simulink model "DOF2_P_SH_ADD_PID_4_0620"  (R2024a)
settings: Solver=ode4  StartTime=0.0  StopTime=10.0  FixedStep=0.001  RelTol=1e-3
undefined symbols (not defined in the file): alpha, badd_AADD, badd_sAADD, cfmax_ONOFF, cfmax_sAADD, cfmax_sAPID, cfmax_sASH, cfmax_SH_ADD, co_AADD, co_APID, co_ASH, co_ONOFF, co_sAADD, co_SaFPID, co_sAPID, co_sASH, co_SH_ADD, cs, csky_ASH, csky_sASH, e_range, ec_range, Famax_AADD, Famax_ASH, Kd, Ki, Kp, ks, kt, ms, mt, Z_Kd, Z_Ki, Z_Kp
settings Model: Creator=1  LastModifiedBy=1
settings DataIOCC: ReturnWorkspaceOutputs=off

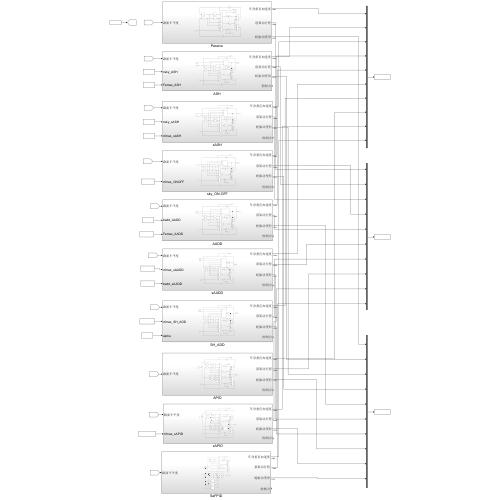
[thumbnail: Simulink's stored preview of the top-level diagram]
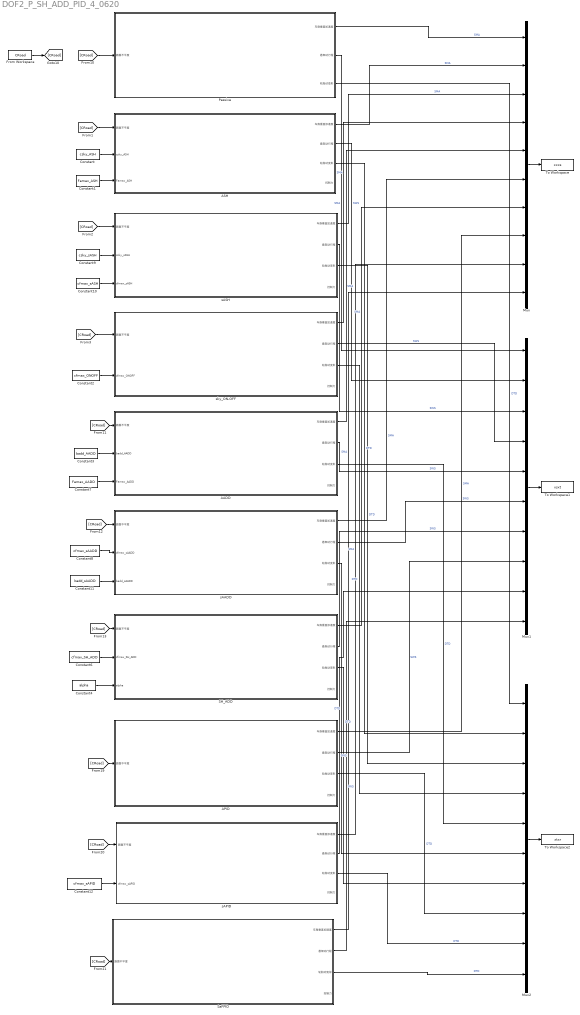
== system DOF2_P_SH_ADD_PID_4_0620 ==
  AADD : Subsystem
  APID : Subsystem
  ASH : Subsystem
  Constant : Constant  Value=csky_ASH
  Constant1 : Constant  Value=Famax_ASH
  Constant10 : Constant  Value=cfmax_sASH
  Constant11 : Constant  Value=badd_sAADD
  Constant12 : Constant  Value=cfmax_sAPID
  Constant2 : Constant  Value=cfmax_ONOFF
  Constant3 : Constant  Value=badd_AADD
  Constant4 : Constant  Value=alpha
  Constant6 : Constant  Value=cfmax_SH_ADD
  Constant7 : Constant  Value=Famax_AADD
  Constant8 : Constant  Value=cfmax_sAADD
  Constant9 : Constant  Value=csky_sASH
  From Workspace : FromWorkspace  VariableName=CRoad
  Mux : Mux  Inputs=10
  Mux1 : Mux  Inputs=10
  Mux2 : Mux  Inputs=10
  Passive : Subsystem
  SH_ADD : Subsystem
  SaFPID : Subsystem
  To Workspace : ToWorkspace  VariableName=xxxs  SampleTime=-1
      settings: Save2DSignal=2-D array (concatenate along first dimension)
  To Workspace1 : ToWorkspace  VariableName=xsxt  SampleTime=-1
      settings: Save2DSignal=2-D array (concatenate along first dimension)
  To Workspace2 : ToWorkspace  VariableName=xtxr  SampleTime=-1
      settings: Save2DSignal=2-D array (concatenate along first dimension)
  sAADD : Subsystem
  sAPID : Subsystem
  sASH : Subsystem
  sky_ON-OFF : Subsystem
  wires:
  From Workspace/1 -> [CRoad]
  [CRoad] -> Passive/1(路面不平度)
  [CRoad] -> ASH/1(路面不平度)
  [CRoad] -> sASH/1(路面不平度)
  [CRoad] -> sky_ON-OFF/1(路面不平度)
  Constant/1 -> ASH/2(csky_ASH)
  Constant9/1 -> sASH/2(csky_sASH)
  Constant1/1 -> ASH/3(Famax_ASH)
  Constant2/1 -> sky_ON-OFF/2(cfmax_ONOFF)
  Mux/1 -> To Workspace/1
  Passive/1(车身垂直加速度) -> Mux/1  "SMA"
  ASH/1(车身垂直加速度) -> Mux/2  "SMA"
  sASH/1(车身垂直加速度) -> Mux/3  "SMA"
  sky_ON-OFF/1(车身垂直加速度) -> Mux/4  "SMA"
  Mux1/1 -> To Workspace1/1
  Passive/2(悬架动行程) -> Mux1/1  "SMA"
  ASH/2(悬架动行程) -> Mux1/2  "SWS"
  sASH/2(悬架动行程) -> Mux1/3  "SWS"
  sky_ON-OFF/2(悬架动行程) -> Mux1/4  "SWS"
  Mux2/1 -> To Workspace2/1
  Passive/3(轮胎动变形) -> Mux2/1  "DTD"
  ASH/3(轮胎动变形) -> Mux2/2  "DTD"
  sASH/3(轮胎动变形) -> Mux2/3  "DTD"
  sky_ON-OFF/3(轮胎动变形) -> Mux2/4  "DTD"
  [CRoad] -> AADD/1(路面不平度)
  [CRoad] -> sAADD/1(路面不平度)
  [CRoad] -> SH_ADD/1(路面不平度)
  Constant7/1 -> AADD/3(Famax_AADD)
  Constant3/1 -> AADD/2(badd_AADD)
  Constant11/1 -> sAADD/3(badd_sAADD)
  Constant4/1 -> SH_ADD/3(alpha)
  AADD/1(车身垂直加速度) -> Mux/5  "SMA"
  sAADD/1(车身垂直加速度) -> Mux/6  "SMA"
  SH_ADD/1(车身垂直加速度) -> Mux/7  "SMA"
  AADD/2(悬架动行程) -> Mux1/5  "SWS"
  sAADD/2(悬架动行程) -> Mux1/6  "SWS"
  SH_ADD/2(悬架动行程) -> Mux1/7  "SWS"
  AADD/3(轮胎动变形) -> Mux2/5  "DTD"
  sAADD/3(轮胎动变形) -> Mux2/6  "DTD"
  SH_ADD/3(轮胎动变形) -> Mux2/7  "DTD"
  Constant6/1 -> SH_ADD/2(cfmax_SH_ADD)
  [CRoad] -> APID/1(路面不平度)
  APID/1(车身垂直加速度) -> Mux/8  "SMA"
  sAPID/1(车身垂直加速度) -> Mux/9  "SMA"
  SaFPID/1(车身垂直加速度) -> Mux/10  "SMA"
  APID/2(悬架动行程) -> Mux1/8  "SWS"
  sAPID/2(悬架动行程) -> Mux1/9  "SWS"
  SaFPID/2(悬架动行程) -> Mux1/10  "SWS"
  APID/3(轮胎动变形) -> Mux2/8  "DTD"
  sAPID/3(轮胎动变形) -> Mux2/9  "DTD"
  SaFPID/3(轮胎动变形) -> Mux2/10  "DTD"
  [CRoad] -> SaFPID/1(路面不平度)
  [CRoad] -> sAPID/1(路面不平度)
  Constant8/1 -> sAADD/2(cfmax_sAADD)
  Constant10/1 -> sASH/3(cfmax_sASH)
  Constant12/1 -> sAPID/2(cfmax_sAPID)

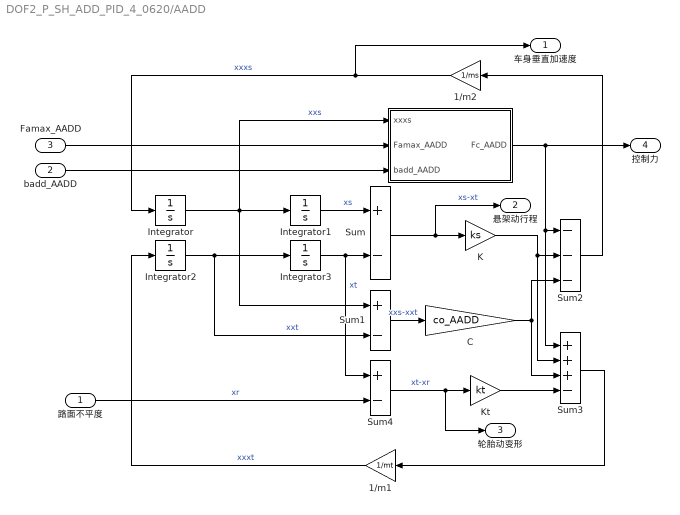
== system DOF2_P_SH_ADD_PID_4_0620/AADD ==
  路面不平度 : Inport
  badd_AADD : Inport  Port=2
  Famax_AADD : Inport  Port=3
  "   " : MATLAB Function  TreatAsAtomicUnit=on
  1/m1 : Gain  Gain=1/mt
  1/m2 : Gain  Gain=1/ms
  C : Gain  Gain=co_AADD
  Integrator{,1..3} (4 alike) : Integrator
  K : Gain  Gain=ks
  "Kt " : Gain  Gain=kt
  Sum : Sum  Inputs=+-
  Sum1 : Sum  Inputs=+-
  Sum2 : Sum  Inputs=---
  Sum3 : Sum  Inputs=+++-
  Sum4 : Sum  Inputs=+-
  车身垂直加速度 : Outport
  悬架动行程 : Outport  Port=2
  轮胎动变形 : Outport  Port=3
  控制力 : Outport  Port=4
  wires:
  Integrator3/1 -> Sum/2, Sum4/1  "xt"
  1/m2/1 -> 车身垂直加速度/1, Integrator/1  "xxxs"
  Integrator/1 -> "   "/1(xxxs), Integrator1/1, Sum1/1  "xxs"
  Sum4/1 -> 轮胎动变形/1, "Kt "/1  "xt-xr"
  Sum1/1 -> C/1  "xxs-xxt"
  Sum2/1 -> 1/m2/1
  Sum/1 -> 悬架动行程/1, K/1  "xs-xt"
  K/1 -> Sum3/2, Sum2/2
  Integrator1/1 -> Sum/1  "xs"
  1/m1/1 -> Integrator2/1  "xxxt"
  Sum3/1 -> 1/m1/1
  Integrator2/1 -> Sum1/2, Integrator3/1  "xxt"
  "Kt "/1 -> Sum3/4
  路面不平度/1 -> Sum4/2  "xr"
  C/1 -> Sum3/3, Sum2/3
  "   "/1(Fc_AADD) -> Sum3/1, Sum2/1, 控制力/1
  badd_AADD/1 -> "   "/3(badd_AADD)
  Famax_AADD/1 -> "   "/2(Famax_AADD)

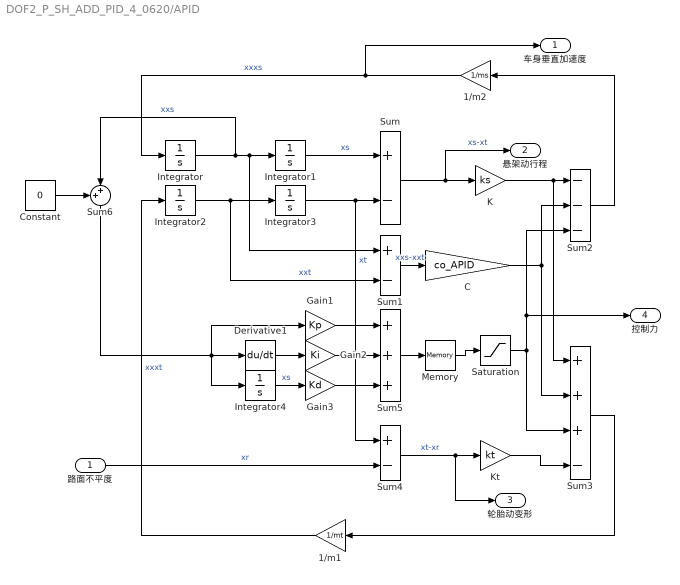
== system DOF2_P_SH_ADD_PID_4_0620/APID ==
  路面不平度 : Inport
  1/m1 : Gain  Gain=1/mt
  1/m2 : Gain  Gain=1/ms
  C : Gain  Gain=co_APID
  Constant : Constant  Value=0
  Derivative1 : Derivative
  Gain1 : Gain  Gain=Kp
  Gain2 : Gain  Gain=Ki
  Gain3 : Gain  Gain=Kd
  Integrator{,1..4} (5 alike) : Integrator
  K : Gain  Gain=ks
  "Kt " : Gain  Gain=kt
  Memory : Memory
  Saturation : Saturate  UpperLimit=2000  LowerLimit=-2000
  Sum : Sum  Inputs=+-
  Sum1 : Sum  Inputs=+-
  Sum2 : Sum  Inputs=---
  Sum3 : Sum  Inputs=+++-
  Sum4 : Sum  Inputs=+-
  Sum5 : Sum  Inputs=+++
  Sum6 : Sum  Inputs=++|
  车身垂直加速度 : Outport
  悬架动行程 : Outport  Port=2
  轮胎动变形 : Outport  Port=3
  控制力 : Outport  Port=4
  wires:
  1/m1/1 -> Integrator2/1  "xxxt"
  Gain2/1 -> Sum5/2
  Sum4/1 -> 轮胎动变形/1, "Kt "/1  "xt-xr"
  Sum6/1 -> Integrator4/1, Gain1/1, Derivative1/1
  Sum2/1 -> 1/m2/1
  Sum1/1 -> C/1  "xxs-xxt"
  Integrator1/1 -> Sum/1  "xs"
  Integrator4/1 -> Gain3/1  "xs"
  Derivative1/1 -> Gain2/1
  Gain1/1 -> Sum5/1
  路面不平度/1 -> Sum4/2  "xr"
  Saturation/1 -> Sum3/3, 控制力/1, Sum2/3
  Sum/1 -> 悬架动行程/1, K/1  "xs-xt"
  C/1 -> Sum2/2, Sum3/2
  Gain3/1 -> Sum5/3
  Integrator3/1 -> Sum/2, Sum4/1  "xt"
  Integrator2/1 -> Sum1/2, Integrator3/1  "xxt"
  1/m2/1 -> 车身垂直加速度/1, Integrator/1  "xxxs"
  K/1 -> Sum3/1, Sum2/1
  Integrator/1 -> Integrator1/1, Sum1/1, Sum6/2  "xxs"
  Sum3/1 -> 1/m1/1
  "Kt "/1 -> Sum3/4
  Sum5/1 -> Memory/1
  Memory/1 -> Saturation/1
  Constant/1 -> Sum6/1

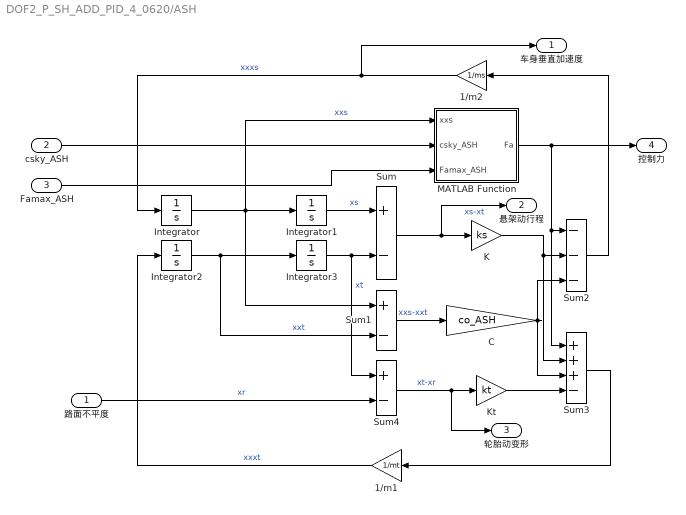
== system DOF2_P_SH_ADD_PID_4_0620/ASH ==
  路面不平度 : Inport
  csky_ASH : Inport  Port=2
  Famax_ASH : Inport  Port=3
  1/m1 : Gain  Gain=1/mt
  1/m2 : Gain  Gain=1/ms
  C : Gain  Gain=co_ASH
  Integrator{,1..3} (4 alike) : Integrator
  K : Gain  Gain=ks
  "Kt " : Gain  Gain=kt
  MATLAB Function : MATLAB Function  TreatAsAtomicUnit=on
  Sum : Sum  Inputs=+-
  Sum1 : Sum  Inputs=+-
  Sum2 : Sum  Inputs=---
  Sum3 : Sum  Inputs=+++-
  Sum4 : Sum  Inputs=+-
  车身垂直加速度 : Outport
  悬架动行程 : Outport  Port=2
  轮胎动变形 : Outport  Port=3
  控制力 : Outport  Port=4
  wires:
  Integrator3/1 -> Sum/2, Sum4/1  "xt"
  1/m2/1 -> 车身垂直加速度/1, Integrator/1  "xxxs"
  Integrator/1 -> MATLAB Function/1(xxs), Integrator1/1, Sum1/1  "xxs"
  Sum4/1 -> 轮胎动变形/1, "Kt "/1  "xt-xr"
  Sum1/1 -> C/1  "xxs-xxt"
  Sum2/1 -> 1/m2/1
  Sum/1 -> 悬架动行程/1, K/1  "xs-xt"
  K/1 -> Sum2/2, Sum3/2
  Integrator1/1 -> Sum/1  "xs"
  1/m1/1 -> Integrator2/1  "xxxt"
  Sum3/1 -> 1/m1/1
  Integrator2/1 -> Sum1/2, Integrator3/1  "xxt"
  "Kt "/1 -> Sum3/4
  路面不平度/1 -> Sum4/2  "xr"
  C/1 -> Sum3/3, Sum2/3
  MATLAB Function/1(Fa) -> Sum3/1, Sum2/1, 控制力/1
  csky_ASH/1 -> MATLAB Function/2(csky_ASH)
  Famax_ASH/1 -> MATLAB Function/3(Famax_ASH)

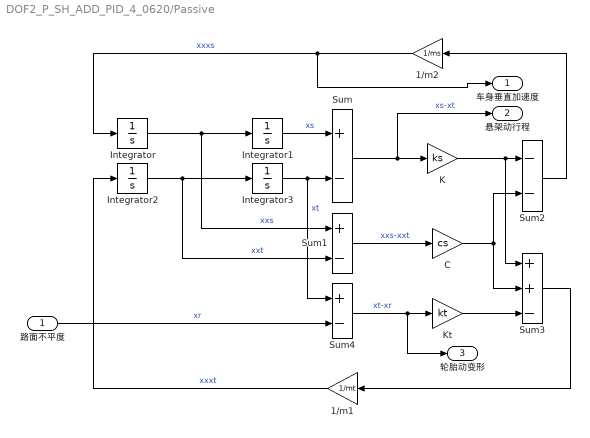
== system DOF2_P_SH_ADD_PID_4_0620/Passive ==
  路面不平度 : Inport
  1/m1 : Gain  Gain=1/mt
  1/m2 : Gain  Gain=1/ms
  C : Gain  Gain=cs
  Integrator{,1..3} (4 alike) : Integrator
  K : Gain  Gain=ks
  "Kt " : Gain  Gain=kt
  Sum : Sum  Inputs=+-
  Sum1 : Sum  Inputs=+-
  Sum2 : Sum  Inputs=--
  Sum3 : Sum  Inputs=++-
  Sum4 : Sum  Inputs=+-
  车身垂直加速度 : Outport
  悬架动行程 : Outport  Port=2
  轮胎动变形 : Outport  Port=3
  wires:
  Integrator3/1 -> Sum/2, Sum4/1  "xt"
  1/m2/1 -> 车身垂直加速度/1, Integrator/1  "xxxs"
  Integrator/1 -> Integrator1/1, Sum1/1  "xxs"
  Sum4/1 -> 轮胎动变形/1, "Kt "/1  "xt-xr"
  Sum1/1 -> C/1  "xxs-xxt"
  Sum2/1 -> 1/m2/1
  Sum/1 -> 悬架动行程/1, K/1  "xs-xt"
  K/1 -> Sum2/1, Sum3/1
  Integrator1/1 -> Sum/1  "xs"
  1/m1/1 -> Integrator2/1  "xxxt"
  Sum3/1 -> 1/m1/1
  Integrator2/1 -> Sum1/2, Integrator3/1  "xxt"
  "Kt "/1 -> Sum3/3
  路面不平度/1 -> Sum4/2  "xr"
  C/1 -> Sum2/2, Sum3/2

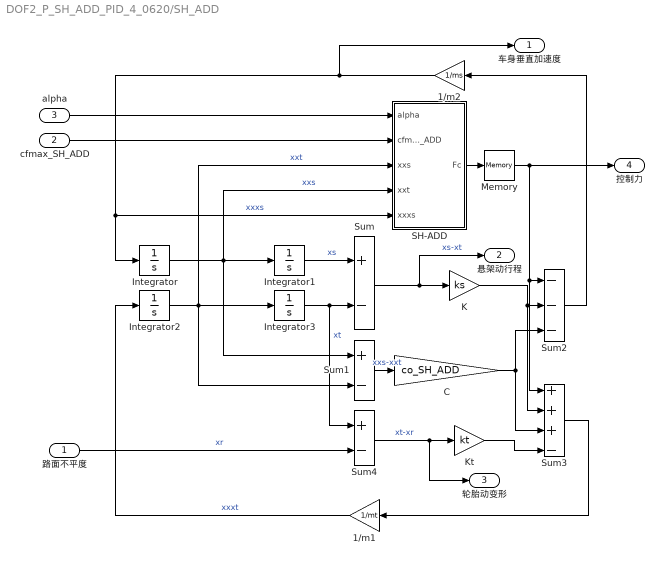
== system DOF2_P_SH_ADD_PID_4_0620/SH_ADD ==
  路面不平度 : Inport
  cfmax_SH_ADD : Inport  Port=2
  alpha : Inport  Port=3
  1/m1 : Gain  Gain=1/mt
  1/m2 : Gain  Gain=1/ms
  C : Gain  Gain=co_SH_ADD
  Integrator{,1..3} (4 alike) : Integrator
  K : Gain  Gain=ks
  "Kt " : Gain  Gain=kt
  Memory : Memory
  SH-ADD : MATLAB Function  TreatAsAtomicUnit=on
  Sum : Sum  Inputs=+-
  Sum1 : Sum  Inputs=+-
  Sum2 : Sum  Inputs=---
  Sum3 : Sum  Inputs=+++-
  Sum4 : Sum  Inputs=+-
  车身垂直加速度 : Outport
  悬架动行程 : Outport  Port=2
  轮胎动变形 : Outport  Port=3
  控制力 : Outport  Port=4
  wires:
  Integrator3/1 -> Sum/2, Sum4/1  "xt"
  1/m2/1 -> 车身垂直加速度/1, SH-ADD/5(xxxs), Integrator/1  "xxxs"
  Integrator/1 -> SH-ADD/4(xxt), Integrator1/1, Sum1/1  "xxs"
  Sum4/1 -> 轮胎动变形/1, "Kt "/1  "xt-xr"
  Sum1/1 -> C/1  "xxs-xxt"
  Sum2/1 -> 1/m2/1
  Sum/1 -> 悬架动行程/1, K/1  "xs-xt"
  K/1 -> Sum2/2, Sum3/2
  Integrator1/1 -> Sum/1  "xs"
  1/m1/1 -> Integrator2/1  "xxxt"
  Sum3/1 -> 1/m1/1
  Integrator2/1 -> SH-ADD/3(xxs), Sum1/2, Integrator3/1  "xxt"
  "Kt "/1 -> Sum3/4
  路面不平度/1 -> Sum4/2  "xr"
  C/1 -> Sum2/3, Sum3/3
  SH-ADD/1(Fc) -> Memory/1
  cfmax_SH_ADD/1 -> SH-ADD/2(cfmax_SH_ADD)
  alpha/1 -> SH-ADD/1(alpha)
  Memory/1 -> Sum3/1, Sum2/1, 控制力/1

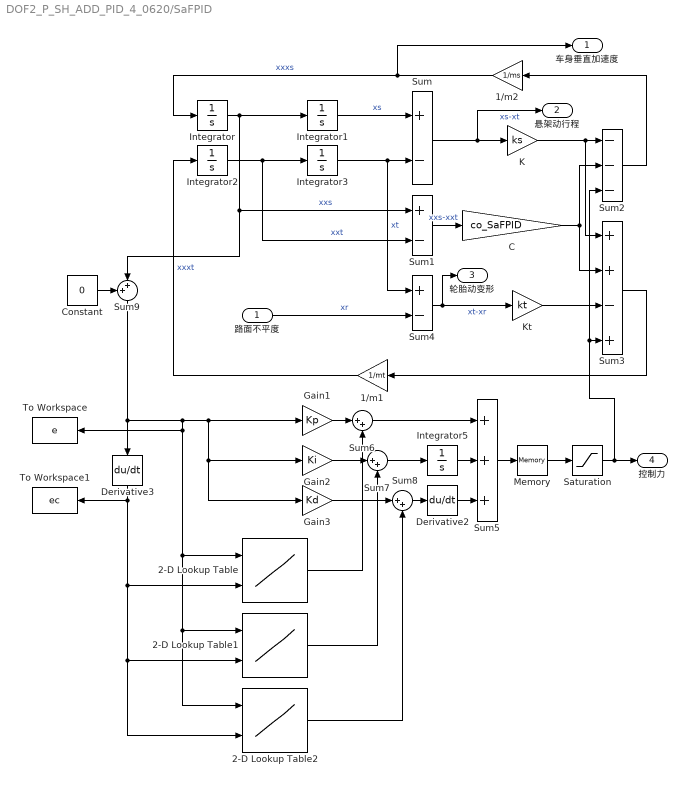
== system DOF2_P_SH_ADD_PID_4_0620/SaFPID ==
  路面不平度 : Inport
  1/m1 : Gain  Gain=1/mt
  1/m2 : Gain  Gain=1/ms
  2-D Lookup Table : Lookup_n-D  BreakpointsForDimension1=e_range  BreakpointsForDimension2=ec_range  Table=Z_Kp  InternalRulePriority=Speed  RndMeth=Simplest
      settings: InputPortMap=u0,u1
  2-D Lookup Table1 : Lookup_n-D  BreakpointsForDimension1=e_range  BreakpointsForDimension2=ec_range  Table=Z_Ki  InternalRulePriority=Speed  RndMeth=Simplest
      settings: InputPortMap=u0,u1
  2-D Lookup Table2 : Lookup_n-D  BreakpointsForDimension1=e_range  BreakpointsForDimension2=ec_range  Table=Z_Kd  InternalRulePriority=Speed  RndMeth=Simplest
      settings: InputPortMap=u0,u1
  C : Gain  Gain=co_SaFPID
  Constant : Constant  Value=0
  Derivative2 : Derivative
  Derivative3 : Derivative
  Gain1 : Gain  Gain=Kp
  Gain2 : Gain  Gain=Ki
  Gain3 : Gain  Gain=Kd
  Integrator{,1..3,5} (5 alike) : Integrator
  K : Gain  Gain=ks
  "Kt " : Gain  Gain=kt
  Memory : Memory
  Saturation : Saturate  UpperLimit=2000  LowerLimit=-2000
  Sum : Sum  Inputs=+-
  Sum1 : Sum  Inputs=+-
  Sum2 : Sum  Inputs=---
  Sum3 : Sum  Inputs=++-+
  Sum4 : Sum  Inputs=+-
  Sum5 : Sum  Inputs=+++
  Sum6 : Sum  Inputs=|++
  Sum7 : Sum  Inputs=|++
  Sum8 : Sum  Inputs=|++
  Sum9 : Sum  Inputs=++|
  To Workspace : ToWorkspace  VariableName=e  SampleTime=-1
      settings: Save2DSignal=2-D array (concatenate along first dimension)
  To Workspace1 : ToWorkspace  VariableName=ec  SampleTime=-1
      settings: Save2DSignal=2-D array (concatenate along first dimension)
  车身垂直加速度 : Outport
  悬架动行程 : Outport  Port=2
  轮胎动变形 : Outport  Port=3
  控制力 : Outport  Port=4
  wires:
  "Kt "/1 -> Sum3/3
  1/m2/1 -> 车身垂直加速度/1, Integrator/1  "xxxs"
  Integrator3/1 -> Sum/2, Sum4/1  "xt"
  Sum9/1 -> Gain3/1, Gain2/1, Gain1/1, 2-D Lookup Table2/1, 2-D Lookup Table1/1, 2-D Lookup Table/1, To Workspace/1, Derivative3/1
  Sum4/1 -> "Kt "/1, 轮胎动变形/1  "xt-xr"
  Sum/1 -> 悬架动行程/1, K/1  "xs-xt"
  Sum1/1 -> C/1  "xxs-xxt"
  路面不平度/1 -> Sum4/2  "xr"
  Sum2/1 -> 1/m2/1
  Integrator2/1 -> Sum1/2, Integrator3/1  "xxt"
  1/m1/1 -> Integrator2/1  "xxxt"
  K/1 -> Sum3/1, Sum2/1
  Sum5/1 -> Memory/1
  C/1 -> Sum2/2, Sum3/2
  Integrator1/1 -> Sum/1  "xs"
  Sum3/1 -> 1/m1/1
  Integrator/1 -> Sum9/2, Sum1/1, Integrator1/1  "xxs"
  Gain1/1 -> Sum6/1
  Gain2/1 -> Sum7/1
  Gain3/1 -> Sum8/1
  Sum6/1 -> Sum5/1
  Sum7/1 -> Integrator5/1
  Integrator5/1 -> Sum5/2
  Sum8/1 -> Derivative2/1
  Derivative2/1 -> Sum5/3
  Saturation/1 -> Sum2/3, Sum3/4, 控制力/1
  Memory/1 -> Saturation/1
  Derivative3/1 -> 2-D Lookup Table2/2, 2-D Lookup Table1/2, 2-D Lookup Table/2, To Workspace1/1
  Constant/1 -> Sum9/1
  2-D Lookup Table/1 -> Sum6/2
  2-D Lookup Table1/1 -> Sum7/2
  2-D Lookup Table2/1 -> Sum8/2

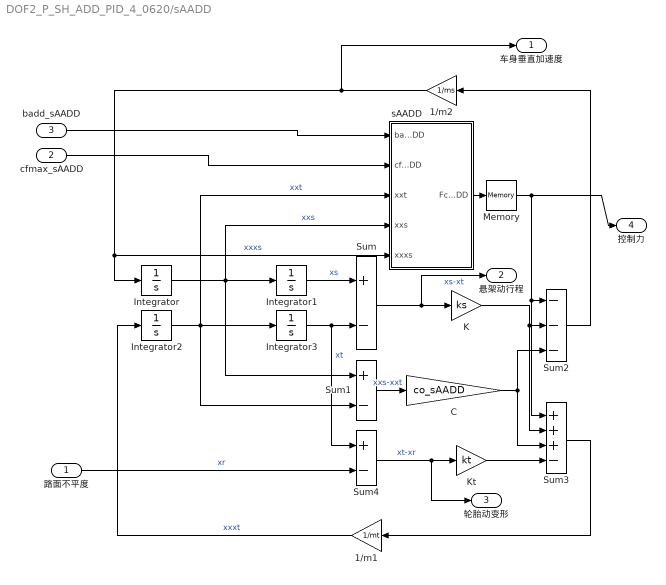
== system DOF2_P_SH_ADD_PID_4_0620/sAADD ==
  路面不平度 : Inport
  cfmax_sAADD : Inport  Port=2
  badd_sAADD : Inport  Port=3
  1/m1 : Gain  Gain=1/mt
  1/m2 : Gain  Gain=1/ms
  C : Gain  Gain=co_sAADD
  Integrator{,1..3} (4 alike) : Integrator
  K : Gain  Gain=ks
  "Kt " : Gain  Gain=kt
  Memory : Memory
  Sum : Sum  Inputs=+-
  Sum1 : Sum  Inputs=+-
  Sum2 : Sum  Inputs=---
  Sum3 : Sum  Inputs=+++-
  Sum4 : Sum  Inputs=+-
  sAADD : MATLAB Function  TreatAsAtomicUnit=on
  车身垂直加速度 : Outport
  悬架动行程 : Outport  Port=2
  轮胎动变形 : Outport  Port=3
  控制力 : Outport  Port=4
  wires:
  Integrator3/1 -> Sum/2, Sum4/1  "xt"
  1/m2/1 -> Integrator/1, sAADD/5(xxxs), 车身垂直加速度/1  "xxxs"
  Integrator/1 -> sAADD/4(xxs), Integrator1/1, Sum1/1  "xxs"
  Sum4/1 -> 轮胎动变形/1, "Kt "/1  "xt-xr"
  Sum1/1 -> C/1  "xxs-xxt"
  Sum/1 -> 悬架动行程/1, K/1  "xs-xt"
  K/1 -> Sum2/2, Sum3/2
  Integrator1/1 -> Sum/1  "xs"
  1/m1/1 -> Integrator2/1  "xxxt"
  Sum3/1 -> 1/m1/1
  Integrator2/1 -> sAADD/3(xxt), Sum1/2, Integrator3/1  "xxt"
  "Kt "/1 -> Sum3/4
  路面不平度/1 -> Sum4/2  "xr"
  C/1 -> Sum2/3, Sum3/3
  Memory/1 -> Sum3/1, Sum2/1, 控制力/1
  cfmax_sAADD/1 -> sAADD/2(cfmax_sAADD)
  badd_sAADD/1 -> sAADD/1(badd_sAADD)
  Sum2/1 -> 1/m2/1
  sAADD/1(Fc_sAADD) -> Memory/1

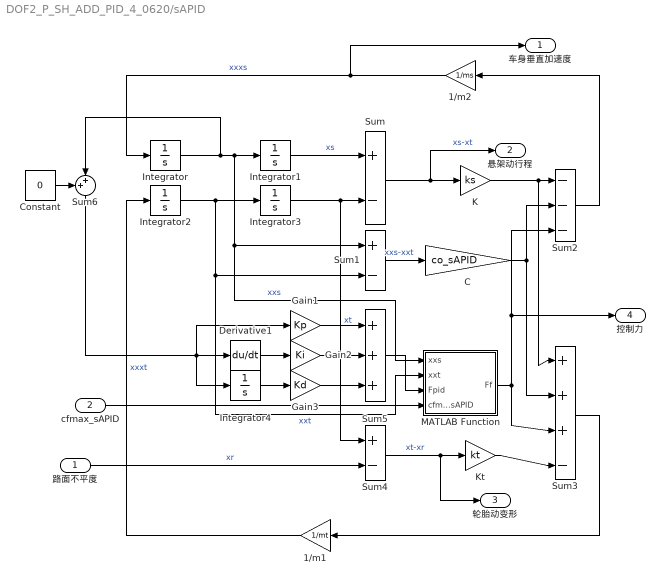
== system DOF2_P_SH_ADD_PID_4_0620/sAPID ==
  路面不平度 : Inport
  cfmax_sAPID : Inport  Port=2
  1/m1 : Gain  Gain=1/mt
  1/m2 : Gain  Gain=1/ms
  C : Gain  Gain=co_sAPID
  Constant : Constant  Value=0
  Derivative1 : Derivative
  Gain1 : Gain  Gain=Kp
  Gain2 : Gain  Gain=Ki
  Gain3 : Gain  Gain=Kd
  Integrator{,1..4} (5 alike) : Integrator
  K : Gain  Gain=ks
  "Kt " : Gain  Gain=kt
  MATLAB Function : MATLAB Function  TreatAsAtomicUnit=on
  Sum : Sum  Inputs=+-
  Sum1 : Sum  Inputs=+-
  Sum2 : Sum  Inputs=---
  Sum3 : Sum  Inputs=+++-
  Sum4 : Sum  Inputs=+-
  Sum5 : Sum  Inputs=+++
  Sum6 : Sum  Inputs=++|
  车身垂直加速度 : Outport
  悬架动行程 : Outport  Port=2
  轮胎动变形 : Outport  Port=3
  控制力 : Outport  Port=4
  wires:
  "Kt "/1 -> Sum3/4
  1/m2/1 -> 车身垂直加速度/1, Integrator/1  "xxxs"
  Integrator3/1 -> Sum/2, Sum4/1  "xt"
  Derivative1/1 -> Gain2/1
  Gain2/1 -> Sum5/2
  Integrator4/1 -> Gain3/1
  Sum4/1 -> 轮胎动变形/1, "Kt "/1  "xt-xr"
  Sum/1 -> 悬架动行程/1, K/1  "xs-xt"
  Sum1/1 -> C/1  "xxs-xxt"
  路面不平度/1 -> Sum4/2  "xr"
  Sum2/1 -> 1/m2/1
  Integrator2/1 -> MATLAB Function/2(xxt), Sum1/2, Integrator3/1  "xxt"
  1/m1/1 -> Integrator2/1  "xxxt"
  K/1 -> Sum3/1, Sum2/1
  MATLAB Function/1(Ff) -> 控制力/1, Sum2/3, Sum3/3
  Sum5/1 -> MATLAB Function/3(Fpid)
  C/1 -> Sum2/2, Sum3/2
  Gain1/1 -> Sum5/1
  Integrator1/1 -> Sum/1  "xs"
  Sum3/1 -> 1/m1/1
  Integrator/1 -> Integrator1/1, MATLAB Function/1(xxs), Sum1/1, Sum6/2  "xxs"
  Gain3/1 -> Sum5/3
  Sum6/1 -> Integrator4/1, Gain1/1, Derivative1/1
  Constant/1 -> Sum6/1
  cfmax_sAPID/1 -> MATLAB Function/4(cfmax_sAPID)

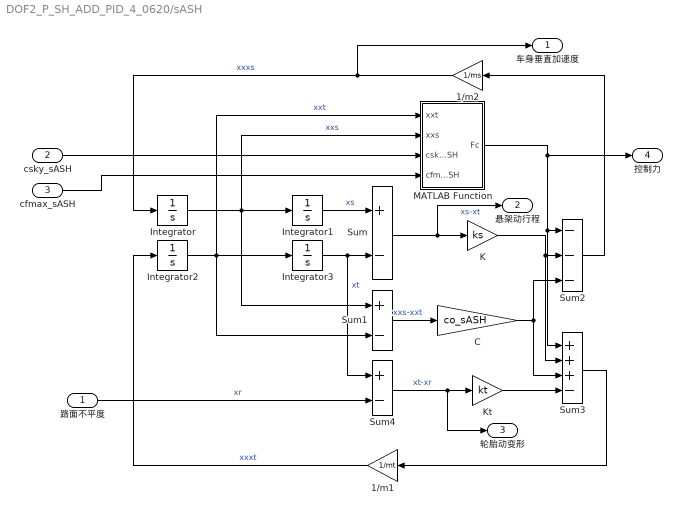
== system DOF2_P_SH_ADD_PID_4_0620/sASH ==
  路面不平度 : Inport
  csky_sASH : Inport  Port=2
  cfmax_sASH : Inport  Port=3
  1/m1 : Gain  Gain=1/mt
  1/m2 : Gain  Gain=1/ms
  C : Gain  Gain=co_sASH
  Integrator{,1..3} (4 alike) : Integrator
  K : Gain  Gain=ks
  "Kt " : Gain  Gain=kt
  MATLAB Function : MATLAB Function  TreatAsAtomicUnit=on
  Sum : Sum  Inputs=+-
  Sum1 : Sum  Inputs=+-
  Sum2 : Sum  Inputs=---
  Sum3 : Sum  Inputs=+++-
  Sum4 : Sum  Inputs=+-
  车身垂直加速度 : Outport
  悬架动行程 : Outport  Port=2
  轮胎动变形 : Outport  Port=3
  控制力 : Outport  Port=4
  wires:
  Integrator3/1 -> Sum/2, Sum4/1  "xt"
  1/m2/1 -> 车身垂直加速度/1, Integrator/1  "xxxs"
  Integrator/1 -> MATLAB Function/2(xxs), Integrator1/1, Sum1/1  "xxs"
  Sum4/1 -> 轮胎动变形/1, "Kt "/1  "xt-xr"
  Sum1/1 -> C/1  "xxs-xxt"
  Sum2/1 -> 1/m2/1
  Sum/1 -> 悬架动行程/1, K/1  "xs-xt"
  K/1 -> Sum3/2, Sum2/2
  Integrator1/1 -> Sum/1  "xs"
  1/m1/1 -> Integrator2/1  "xxxt"
  Sum3/1 -> 1/m1/1
  Integrator2/1 -> MATLAB Function/1(xxt), Sum1/2, Integrator3/1  "xxt"
  "Kt "/1 -> Sum3/4
  路面不平度/1 -> Sum4/2  "xr"
  C/1 -> Sum3/3, Sum2/3
  MATLAB Function/1(Fc) -> Sum3/1, Sum2/1, 控制力/1
  csky_sASH/1 -> MATLAB Function/3(csky_sASH)
  cfmax_sASH/1 -> MATLAB Function/4(cfmax_sASH)

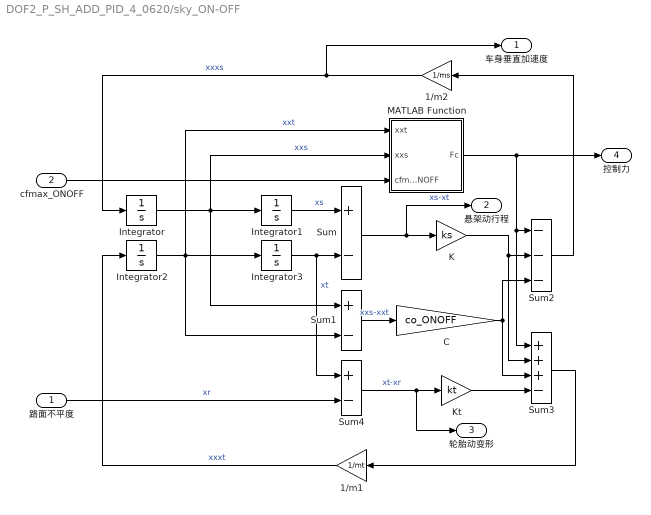
== system DOF2_P_SH_ADD_PID_4_0620/sky_ON-OFF ==
  路面不平度 : Inport
  cfmax_ONOFF : Inport  Port=2
  1/m1 : Gain  Gain=1/mt
  1/m2 : Gain  Gain=1/ms
  C : Gain  Gain=co_ONOFF
  Integrator{,1..3} (4 alike) : Integrator
  K : Gain  Gain=ks
  "Kt " : Gain  Gain=kt
  MATLAB Function : MATLAB Function  TreatAsAtomicUnit=on
  Sum : Sum  Inputs=+-
  Sum1 : Sum  Inputs=+-
  Sum2 : Sum  Inputs=---
  Sum3 : Sum  Inputs=+++-
  Sum4 : Sum  Inputs=+-
  车身垂直加速度 : Outport
  悬架动行程 : Outport  Port=2
  轮胎动变形 : Outport  Port=3
  控制力 : Outport  Port=4
  wires:
  Integrator3/1 -> Sum/2, Sum4/1  "xt"
  1/m2/1 -> 车身垂直加速度/1, Integrator/1  "xxxs"
  Integrator/1 -> MATLAB Function/2(xxs), Integrator1/1, Sum1/1  "xxs"
  Sum4/1 -> 轮胎动变形/1, "Kt "/1  "xt-xr"
  Sum1/1 -> C/1  "xxs-xxt"
  Sum2/1 -> 1/m2/1
  Sum/1 -> 悬架动行程/1, K/1  "xs-xt"
  K/1 -> Sum2/2, Sum3/2
  Integrator1/1 -> Sum/1  "xs"
  1/m1/1 -> Integrator2/1  "xxxt"
  Sum3/1 -> 1/m1/1
  Integrator2/1 -> MATLAB Function/1(xxt), Sum1/2, Integrator3/1  "xxt"
  "Kt "/1 -> Sum3/4
  路面不平度/1 -> Sum4/2  "xr"
  C/1 -> Sum3/3, Sum2/3
  MATLAB Function/1(Fc) -> Sum3/1, Sum2/1, 控制力/1
  cfmax_ONOFF/1 -> MATLAB Function/3(cfmax_ONOFF)

== matlab function DOF2_P_SH_ADD_PID_4_0620/sky_ON-OFF/MATLAB Function ==
  data: xxt input; xxs input; Fc output; cfmax_ONOFF input
function Fc = fcn(xxt, xxs, cfmax_ONOFF)
if xxs*(xxs-xxt)>0
    cf = cfmax_ONOFF;
else
    cf = 0;
end
Fc = cf * (xxs-xxt);

== matlab function DOF2_P_SH_ADD_PID_4_0620/sASH/MATLAB Function ==
  data: xxt input; xxs input; Fc output; csky_sASH input; cfmax_sASH input
function Fc = fcn(xxt, xxs, csky_sASH,cfmax_sASH)
if csky_sASH*xxs/(xxs-xxt)>cfmax_sASH
    cf = cfmax_sASH;
elseif csky_sASH*xxs/(xxs-xxt)>0&&csky_sASH*xxs/(xxs-xxt)<=cfmax_sASH 
        cf = csky_sASH*xxs/(xxs-xxt);
else
    cf = 0;
end
Fc = cf * (xxs-xxt);

== matlab function DOF2_P_SH_ADD_PID_4_0620/ASH/MATLAB Function ==
  data: xxs input; csky_ASH input; Famax_ASH input; Fa output
function Fa = fcn(xxs, csky_ASH, Famax_ASH)
if csky_ASH*xxs>Famax_ASH
    Fa = Famax_ASH;
elseif csky_ASH*xxs>-1*Famax_ASH&&csky_ASH*xxs<=Famax_ASH 
        Fa = csky_ASH*xxs;
else
    Fa = -1*Famax_ASH;
end

== matlab function DOF2_P_SH_ADD_PID_4_0620/SH_ADD/SH-ADD ==
  data: alpha input; cfmax_SH_ADD input; xxs input; Fc output; xxt input; xxxs input
function Fc = fcn(alpha,cfmax_SH_ADD,xxs,xxt,xxxs)
if (((xxxs*xxxs-alpha*alpha*xxs*xxs)<=0)&&(xxs*(xxs-xxt)>0))||(((xxxs*xxxs-alpha*alpha*xxs*xxs)>0)&&(xxxs*(xxs-xxt)>0))
    cf = cfmax_SH_ADD;
else
    cf = 0;
end
Fc = cf*(xxs-xxt);

== matlab function DOF2_P_SH_ADD_PID_4_0620/sAPID/MATLAB Function ==
  data: xxs input; Ff output; xxt input; Fpid input; cfmax_sAPID input
%%% "Ff = sAPID(xxs,xxt,Fpid)" %%%
% 半主动 PID 控制律

function Ff = sAPID(xxs, xxt, Fpid,cfmax_sAPID)
   
    Ff = zeros(size(Fpid)); % 初始化 Ff，确保维度正确

    % 防止除以零的情况
    delta_x = xxs - xxt;
    small_value = 1e-6; % 设定一个很小的值，防止除零
    delta_x(abs(delta_x) < small_value) = small_value;

    % 计算理想情况下的可调阻尼
    cf = Fpid ./ delta_x;

    % 处理不同情况
    for i = 1:numel(Fpid)
        if cf(i) > cfmax_sAPID
            cf(i) = cfmax_sAPID; % 施加最大阻尼
        elseif Fpid(i) * delta_x(i) <= 0
            cf(i) = 0; % 施加最小阻尼
        end
    end

    % 计算最终控制力
    Ff = cf .* delta_x;
end

== matlab function DOF2_P_SH_ADD_PID_4_0620/AADD/    ==
  data: xxxs input; Famax_AADD input; Fc_AADD output; badd_AADD input
function Fc_AADD = AADD(xxxs,Famax_AADD,badd_AADD)
if badd_AADD*xxxs>Famax_AADD
    Fc_AADD = Famax_AADD;
elseif badd_AADD*xxxs<=Famax_AADD&&badd_AADD*xxxs>(-1*Famax_AADD)
    Fc_AADD = badd_AADD*xxxs;
else
    Fc_AADD = -1*Famax_AADD;
end

== matlab function DOF2_P_SH_ADD_PID_4_0620/sAADD/sAADD ==
  data: badd_sAADD input; cfmax_sAADD input; xxt input; xxs input; Fc_sAADD output; xxxs input
function Fc_sAADD = fcn(badd_sAADD,cfmax_sAADD,xxt,xxs,xxxs)
if badd_sAADD*xxxs/(xxs-xxt)> cfmax_sAADD
    cf = cfmax_sAADD;
elseif badd_sAADD*xxxs/(xxs-xxt)<= cfmax_sAADD&&badd_sAADD*xxxs/(xxs-xxt)>0
    cf = badd_sAADD*xxxs/(xxs-xxt);
else
    cf = 0;
end
Fc_sAADD = cf*(xxs-xxt);
